simulink model "sampleModel1480"  (R2023a)
settings: Solver=VariableStepAuto  StartTime=0.0  StopTime=10.0  RelTol=1e-3
libraries: hdlsllib x4, simulink x3
settings Model: Creator=user1  LastModifiedBy=user1

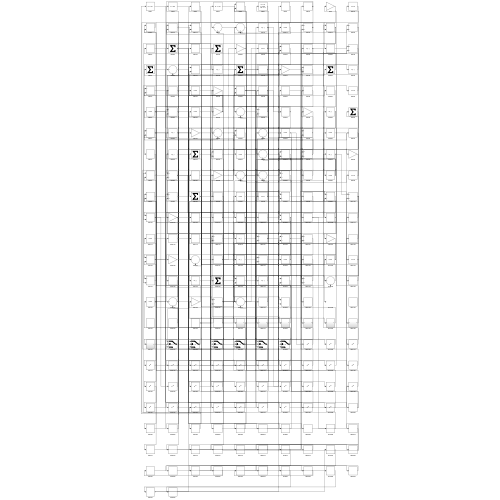
[thumbnail: Simulink's stored preview of the top-level diagram]
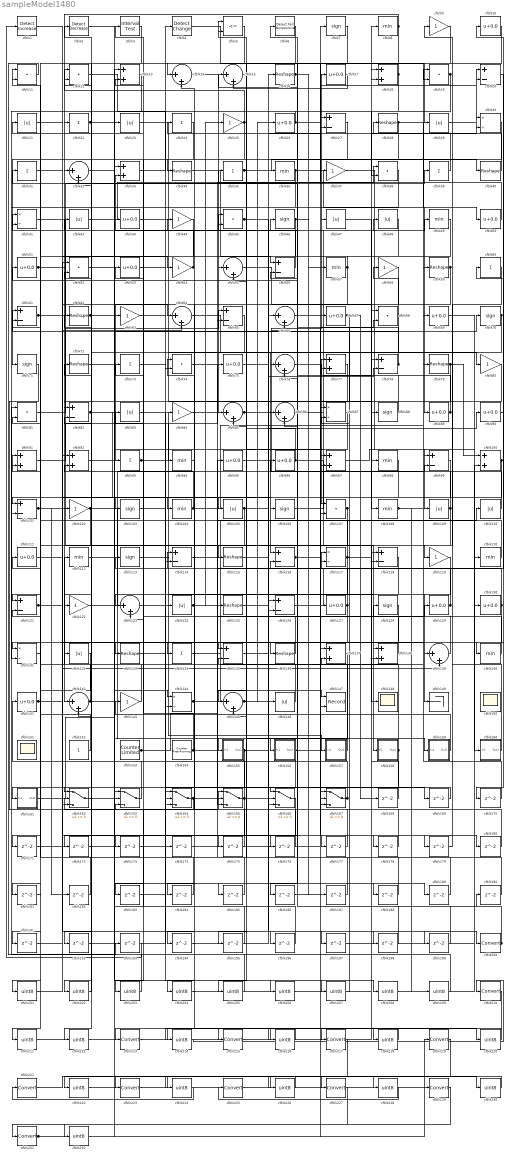
== system sampleModel1480 ==
  cfblk1 : simulink/Logic and Bit Operations/Detect Increase  vinit=0.0  OutDataTypeStr=boolean
      settings: LibrarySourceBlock=|
      | hdlsllib/Logic and Bit
      | Operations/Detect
      | Increase
  cfblk{10,17,26,43,50..51,53,67,69,75,89..90,95..96,111,127,129..130,141} (19 alike) : Bias  Bias=0.0  SaturateOnIntegerOverflow=off
  cfblk{13,18,33,77,91..92,97,100,137..138} (10 alike) : Sum
  cfblk{20,27,56,61,65,78,82,99,101,114,116,118,121,126,135} (15 alike) : Sum  Inputs=+-
  cfblk{9,25,37,44,54,58,63,80,84,102,119,122,143} (13 alike) : Gain
  cfblk{7,46,70..71,88,103,106,113,128} (9 alike) : Signum
  cfblk{8,36,49,57,94,98,104,108,112,120,140} (11 alike) : MinMax
  cfblk{21,23,29,42,47..48,83,105,109..110,124,132,146} (13 alike) : Abs  SaturateOnIntegerOverflow=off
  cfblk{11..12,19,38,45,52,68,74,81,107} (10 alike) : DotProduct  OutDataTypeStr=Inherit: Inherit via internal rule
  cfblk{16,28,34,40,59,62,72,79,115,125,133,136} (12 alike) : Reshape
  cfblk{30,41,87,117,131,144} (6 alike) : Product  Inputs=*/  RndMeth=Zero  SaturateOnIntegerOverflow=on
  cfblk{14..15,32,55,64,66,76,85..86,123,139,142,145} (13 alike) : Sum  Inputs=|++
  cfblk{22,24,31,35,39,60,73,93,134} (9 alike) : Sum  Inputs=+
  cfblk147 : Record  FileSettingsInternal="{\"entries\":[{\"content\":{\"excelSettings\":{\"content\":{},\"type\":\"Streamout.ExcelSettings\"}},\"type\":\"Streamout.FileSettingStorage\",\"uuid\":\"\"}],\"packageUris\":[\"http:\\/\\/schema.mathworks.com\\/mf0\\/streamout_blocks\\/R2020a\"],\"version\":\"1.0\"}"  Layout=[1 1]  SignalsInternal="{\"entries\":[{\"content\":{\"signals\":[{\"content\":{\"blockPath\":[],\"dimensions\":[1],\"domain\":\"\",\"lineColor\":\"#a2142f\",\"plots\":[1],\"port\":1,\"signalID\":1091,\"signalName\":\"XY Graph:1\"},\"type\":\"RecordBlkView.Signal\",\"uuid\":\"\"},{\"content\":{\"blockPath\":[],\"dimensions\":[1],\"domain\":\"\",\"lineColor\":\"#139fff\",\"plots\":[1],\"port\":2,\"signalID\":1094,\"signalName\":\"XY Graph:2\"},\"type\":\"RecordBlkView.Signal\",\"uuid\":\"\"}]},\"type\":\"RecordBlkView.InputSignals\",\"uuid\":\"\"}],\"packageUris\":[\"http:\\/\\/schema.mathworks.com\\/mf0\\/streamout_blocks\\/R2020a\"],\"version\":\"1.0\"}"  VisualizationBindings="{\"xyplotplugin\":{\"info\":[{\"series\":[{\"bindingParametersList\":[{\"parameter\":\"X-Axis\",\"signalID\":1091,\"signalName\":\"XY Graph:1\"},{\"parameter\":\"Y-Axis\",\"signalID\":1094,\"signalName\":\"XY Graph:2\"}],\"seriesID\":44027}],\"subplotID\":1}]}}"  CompatibilityTag=XY  st=-1
  cfblk148 : Scope
  cfblk149 : Terminator
  cfblk150 : Scope
      settings: Floating=on
  cfblk151 : Scope
      settings: Floating=on
  cfblk152 : Constant  SampleTime=-1
  cfblk153 : hdlsllib/Sources/Counter Limited  uplimit=7  tsamp=-1
  cfblk154 : hdlsllib/Sources/Counter Free-Running  NumBits=16  tsamp=-1
  cfblk155 : Subsystem
      settings: LibrarySourceBlock=|
      | hdlsllib/Ports &
      | Subsystems/Subsystem
  cfblk156 : Subsystem
      settings: LibrarySourceBlock=|
      | hdlsllib/Ports &
      | Subsystems/Subsystem
  cfblk157 : Subsystem
      settings: LibrarySourceBlock=|
      | hdlsllib/Ports &
      | Subsystems/Subsystem
  cfblk158 : Subsystem
      settings: LibrarySourceBlock=|
      | hdlsllib/Ports &
      | Subsystems/Subsystem
  cfblk159 : Subsystem
      settings: LibrarySourceBlock=|
      | hdlsllib/Ports &
      | Subsystems/Subsystem
  cfblk160 : Subsystem
      settings: LibrarySourceBlock=|
      | hdlsllib/Ports &
      | Subsystems/Subsystem
  cfblk161 : Subsystem
      settings: LibrarySourceBlock=|
      | hdlsllib/Ports &
      | Subsystems/Subsystem
  cfblk{162..167} (6 alike) : Switch  SaturateOnIntegerOverflow=off  InputSameDT=off
  cfblk{168..199} (32 alike) : Delay  SampleTime=1
  cfblk2 : simulink/Logic and Bit Operations/Detect Decrease  vinit=0.0  OutDataTypeStr=boolean
      settings: LibrarySourceBlock=|
      | hdlsllib/Logic and Bit
      | Operations/Detect
      | Decrease
  cfblk{200,210,213,215,217,219,221,223,225,227,229,231} (12 alike) : DataTypeConversion  SaturateOnIntegerOverflow=off  RndMeth=Floor
  cfblk{201..209,211..212,214,216,218,220,222,224,226,228,230,232} (21 alike) : DataTypeConversion  OutDataTypeStr=uint8  SaturateOnIntegerOverflow=off  RndMeth=Floor
  cfblk3 : hdlsllib/Logic and Bit Operations/Interval Test  IntervalClosedRight=on  uplimit=0.5  IntervalClosedLeft=on  lowlimit=-0.5  OutDataTypeStr=boolean
  cfblk4 : simulink/Logic and Bit Operations/Detect Change  vinit=0  OutDataTypeStr=boolean
      settings: LibrarySourceBlock=|
      | hdlsllib/Logic and Bit
      | Operations/Detect
      | Change
  cfblk5 : RelationalOperator  Operator=<=  OutDataTypeStr=boolean  InputSameDT=off
  cfblk6 : hdlsllib/Logic and Bit Operations/Detect Fall Nonpositive  vinit=0  OutDataTypeStr=boolean
  wires:
  cfblk58/1 -> cfblk93/1
  cfblk102/1 -> cfblk155/1(In1), cfblk121/1
  cfblk105/1 -> cfblk90/1, cfblk197/1, cfblk204/1
  cfblk14/1 -> cfblk85/1
  cfblk83/1 -> cfblk157/1(In1)
  cfblk9/1 -> cfblk29/1
  cfblk82/1 -> cfblk104/1, cfblk159/1(In1)
  cfblk95/1 -> cfblk17/1
  cfblk66/1 -> cfblk47/1
  cfblk97/1 -> cfblk109/1
  cfblk163/1 -> cfblk141/1
  cfblk36/1 -> cfblk89/1, cfblk131/2
  cfblk88/1 -> cfblk15/1
  cfblk8/1 -> cfblk142/1, cfblk147/2
  cfblk144/1 -> cfblk28/1, cfblk68/1, cfblk69/1
  cfblk138/1 -> cfblk21/1
  cfblk126/1 -> cfblk10/1
  cfblk10/1 -> cfblk75/1
  cfblk104/1 -> cfblk79/1, cfblk12/2
  cfblk37/1 -> cfblk160/1(In1)
  cfblk24/1 -> cfblk71/1
  cfblk162/1 -> cfblk23/1
  cfblk158/1(Out1) -> cfblk121/2, cfblk176/1
  cfblk125/1 -> cfblk16/1
  cfblk136/1 -> cfblk83/1
  cfblk63/1 -> cfblk124/1
  cfblk153/1 -> cfblk84/1, cfblk95/1
  cfblk64/1 -> cfblk116/1
  cfblk56/1 -> cfblk11/1
  cfblk17/1 -> cfblk15/2
  cfblk81/1 -> cfblk65/1
  cfblk127/1 -> cfblk5/1, cfblk166/1, cfblk76/2
  cfblk34/1 -> cfblk56/1
  cfblk152/1 -> cfblk11/2
  cfblk77/1 -> cfblk115/1
  cfblk142/1 -> cfblk112/1, cfblk72/1, cfblk198/1
  cfblk101/1 -> cfblk158/1(In1), cfblk182/1
  cfblk71/1 -> cfblk165/1
  cfblk23/1 -> cfblk80/1
  cfblk86/1 -> cfblk49/1
  cfblk124/1 -> cfblk117/1, cfblk25/1
  cfblk100/1 -> cfblk131/1, cfblk170/1
  cfblk112/1 -> cfblk66/2
  cfblk159/1(Out1) -> cfblk143/1
  cfblk130/1 -> cfblk73/1, cfblk186/1
  cfblk84/1 -> cfblk65/2
  cfblk114/1 -> cfblk110/1
  cfblk6/1 -> cfblk32/1
  cfblk50/1 -> cfblk35/1
  cfblk40/1 -> cfblk9/1
  cfblk57/1 -> cfblk55/1, cfblk74/2
  cfblk78/1 -> cfblk61/1, cfblk42/1
  cfblk74/1 -> cfblk147/1
  cfblk93/1 -> cfblk48/1, cfblk133/1
  cfblk85/1 -> cfblk77/1, cfblk139/1
  cfblk92/1 -> cfblk70/1
  cfblk134/1 -> cfblk8/1
  cfblk48/1 -> cfblk101/1
  cfblk7/1 -> cfblk136/1
  cfblk160/1(Out1) -> cfblk24/1
  cfblk157/1(Out1) -> cfblk114/1
  cfblk33/1 -> cfblk4/1
  cfblk28/1 -> cfblk50/1, cfblk173/1
  cfblk43/1 -> cfblk108/1
  cfblk69/1 -> cfblk130/1
  cfblk103/1 -> cfblk156/1(In1)
  cfblk113/1 -> cfblk138/1
  cfblk41/1 -> cfblk125/1
  cfblk161/1(Out1) -> cfblk13/1
  cfblk20/1 -> cfblk140/1
  cfblk80/1 -> cfblk82/1
  cfblk108/1 -> cfblk30/2, cfblk209/1
  cfblk164/1 -> cfblk162/2, cfblk129/1, cfblk74/1
  cfblk18/1 -> cfblk14/1, cfblk107/2
  cfblk59/1 -> cfblk134/1, cfblk166/2
  cfblk46/1 -> cfblk145/2, cfblk187/1
  cfblk122/1 -> cfblk59/1
  cfblk116/1 -> cfblk96/1, cfblk178/1
  cfblk12/1 -> cfblk94/1
  cfblk87/1 -> cfblk135/1
  cfblk61/1 -> cfblk7/1, cfblk199/1
  cfblk4/1 -> cfblk19/2
  cfblk155/1(Out1) -> cfblk128/1, cfblk191/1
  cfblk47/1 -> cfblk99/1
  cfblk31/1 -> cfblk54/1
  cfblk96/1 -> cfblk148/1, cfblk45/1
  cfblk22/1 -> cfblk97/1, cfblk189/1
  cfblk143/1 -> cfblk91/1
  cfblk67/1 -> cfblk87/1, cfblk168/1
  cfblk35/1 -> cfblk40/1, cfblk27/2
  cfblk156/1(Out1) -> cfblk164/2, cfblk68/2
  cfblk120/1 -> cfblk81/2
  cfblk121/1 -> cfblk64/2, cfblk177/1
  cfblk26/1 -> cfblk22/1, cfblk20/2
  cfblk129/1 -> cfblk123/1, cfblk113/1
  cfblk45/1 -> cfblk97/2, cfblk179/1, cfblk180/1
  cfblk68/1 -> cfblk58/1, cfblk76/1
  cfblk90/1 -> cfblk60/1
  cfblk75/1 -> cfblk36/1
  cfblk42/1 -> cfblk38/1
  cfblk115/1 -> cfblk78/2
  cfblk135/1 -> cfblk126/2
  cfblk131/1 -> cfblk41/1
  cfblk91/1 -> cfblk37/1
  cfblk25/1 -> cfblk34/1, cfblk12/1
  cfblk51/1 -> cfblk39/1, cfblk139/2
  cfblk167/1 -> cfblk62/1, cfblk6/1
  cfblk140/1 -> cfblk53/1
  cfblk15/1 -> cfblk105/1
  cfblk89/1 -> cfblk31/1, cfblk51/1, cfblk56/2
  cfblk21/1 -> cfblk64/1
  cfblk106/1 -> cfblk18/2
  cfblk60/1 -> cfblk119/1
  cfblk154/1 -> cfblk116/2, cfblk13/2
  cfblk141/1 -> cfblk92/1, cfblk196/1
  cfblk110/1 -> cfblk67/1
  cfblk13/1 -> cfblk101/2
  cfblk54/1 -> cfblk33/2, cfblk3/1
  cfblk16/1 -> cfblk86/1, cfblk57/1
  cfblk165/1 -> cfblk146/1, cfblk27/1, cfblk111/1, cfblk192/1
  cfblk111/1 -> cfblk138/2
  cfblk29/1 -> cfblk20/1
  cfblk27/1 -> cfblk32/2
  cfblk145/1 -> cfblk26/1, cfblk188/1
  cfblk52/1 -> cfblk200/1
  cfblk5/1 -> cfblk161/1(In1)
  cfblk119/1 -> cfblk149/1
  cfblk1/1 -> cfblk106/1
  cfblk62/1 -> cfblk144/1, cfblk102/1, cfblk45/2
  cfblk139/1 -> cfblk44/1
  cfblk79/1 -> cfblk123/2, cfblk100/1
  cfblk44/1 -> cfblk164/3
  cfblk19/1 -> cfblk38/2, cfblk145/1
  cfblk30/1 -> cfblk167/2
  cfblk109/1 -> cfblk132/1, cfblk86/2
  cfblk117/1 -> cfblk165/3, cfblk91/2, cfblk30/1
  cfblk146/1 -> cfblk43/1
  cfblk76/1 -> cfblk107/1
  cfblk55/1 -> cfblk88/1
  cfblk107/1 -> cfblk166/3, cfblk183/1
  cfblk70/1 -> cfblk195/1, cfblk212/1
  cfblk39/1 -> cfblk5/2
  cfblk99/1 -> cfblk103/1
  cfblk38/1 -> cfblk122/1
  cfblk168/1 -> cfblk18/1
  cfblk123/1 -> cfblk169/1
  cfblk169/1 -> cfblk162/1
  cfblk170/1 -> cfblk19/1
  cfblk49/1 -> cfblk171/1
  cfblk171/1 -> cfblk126/1
  cfblk65/1 -> cfblk172/1
  cfblk172/1 -> cfblk92/2
  cfblk173/1 -> cfblk164/1
  cfblk53/1 -> cfblk174/1
  cfblk174/1 -> cfblk117/2
  cfblk32/1 -> cfblk175/1
  cfblk175/1 -> cfblk142/2
  cfblk176/1 -> cfblk33/1
  cfblk177/1 -> cfblk135/2
  cfblk178/1 -> cfblk78/1
  cfblk179/1 -> cfblk99/2
  cfblk180/1 -> cfblk14/2
  cfblk132/1 -> cfblk181/1
  cfblk182/1 -> cfblk41/2
  cfblk183/1 -> cfblk144/2
  cfblk166/1 -> cfblk184/1
  cfblk184/1 -> cfblk82/2
  cfblk73/1 -> cfblk185/1
  cfblk185/1 -> cfblk61/2
  cfblk186/1 -> cfblk167/3
  cfblk187/1 -> cfblk167/1
  cfblk188/1 -> cfblk85/2
  cfblk189/1 -> cfblk165/2
  cfblk190/1 -> cfblk55/2
  cfblk191/1 -> cfblk162/3
  cfblk192/1 -> cfblk114/2
  cfblk11/1 -> cfblk193/1
  cfblk193/1 -> cfblk1/1
  cfblk94/1 -> cfblk194/1
  cfblk194/1 -> cfblk66/1
  cfblk195/1 -> cfblk163/2
  cfblk196/1 -> cfblk163/3
  cfblk197/1 -> cfblk100/2
  cfblk198/1 -> cfblk87/2
  cfblk199/1 -> cfblk77/2
  cfblk200/1 -> cfblk190/1, cfblk46/1
  cfblk128/1 -> cfblk201/1
  cfblk201/1 -> cfblk52/1
  cfblk3/1 -> cfblk202/1
  cfblk202/1 -> cfblk52/2
  cfblk98/1 -> cfblk203/1
  cfblk203/1 -> cfblk163/1
  cfblk204/1 -> cfblk98/1
  cfblk137/1 -> cfblk205/1
  cfblk205/1 -> cfblk81/1
  cfblk133/1 -> cfblk206/1
  cfblk206/1 -> cfblk137/1
  cfblk72/1 -> cfblk207/1
  cfblk207/1 -> cfblk137/2
  cfblk2/1 -> cfblk208/1
  cfblk208/1 -> cfblk120/1
  cfblk209/1 -> cfblk2/1
  cfblk181/1 -> cfblk211/1
  cfblk211/1 -> cfblk118/1
  cfblk212/1 -> cfblk118/2
  cfblk118/1 -> cfblk214/1
  cfblk214/1 -> cfblk210/1
  cfblk210/1 -> cfblk216/1
  cfblk216/1 -> cfblk213/1
  cfblk213/1 -> cfblk218/1
  cfblk218/1 -> cfblk215/1
  cfblk215/1 -> cfblk220/1
  cfblk220/1 -> cfblk217/1
  cfblk217/1 -> cfblk222/1
  cfblk222/1 -> cfblk219/1
  cfblk219/1 -> cfblk224/1
  cfblk224/1 -> cfblk221/1
  cfblk221/1 -> cfblk226/1
  cfblk226/1 -> cfblk223/1
  cfblk223/1 -> cfblk228/1
  cfblk228/1 -> cfblk225/1
  cfblk229/1 -> cfblk231/1
  cfblk225/1 -> cfblk230/1
  cfblk230/1 -> cfblk227/1
  cfblk231/1 -> cfblk127/1, cfblk63/1
  cfblk227/1 -> cfblk232/1
  cfblk232/1 -> cfblk229/1

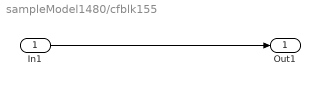
== system sampleModel1480/cfblk155 ==
  In1 : Inport
  Out1 : Outport
  wires:
  In1/1 -> Out1/1

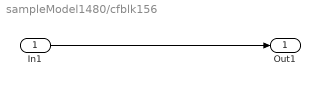
== system sampleModel1480/cfblk156 ==
  In1 : Inport
  Out1 : Outport
  wires:
  In1/1 -> Out1/1

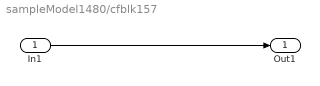
== system sampleModel1480/cfblk157 ==
  In1 : Inport
  Out1 : Outport
  wires:
  In1/1 -> Out1/1

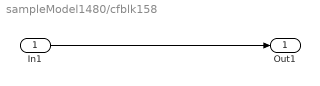
== system sampleModel1480/cfblk158 ==
  In1 : Inport
  Out1 : Outport
  wires:
  In1/1 -> Out1/1

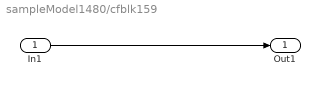
== system sampleModel1480/cfblk159 ==
  In1 : Inport
  Out1 : Outport
  wires:
  In1/1 -> Out1/1

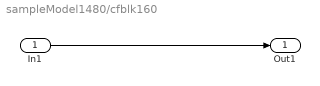
== system sampleModel1480/cfblk160 ==
  In1 : Inport
  Out1 : Outport
  wires:
  In1/1 -> Out1/1

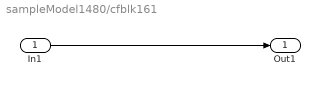
== system sampleModel1480/cfblk161 ==
  In1 : Inport
  Out1 : Outport
  wires:
  In1/1 -> Out1/1
